simulink model "Concatenate9"  (R2017b)
settings: Solver=FixedStepAuto  StartTime=0.0  StopTime=0  FixedStep=0.1  MaxStep=1  RelTol=1e-3  EnableMultiTasking=on
settings Model: Creator=arnaud  LastModifiedBy=hbourbou
settings DataIOCC: LimitDataPoints=on  SaveFormat=Structure
settings OptimizationCC: LifeSpan=inf
settings DebuggingCC: SolverPrmCheckMsg=warning  SFUnexpectedBacktrackingDiag=warning  SFNoUnconditionalDefaultTransitionDiag=warning  SFExecutionAtInitializationDiag=none
settings HardwareCC: ProdBitPerPointer=32  ProdBitPerSizeT=32  ProdBitPerPtrDiffT=32  ProdLargestAtomicFloat=None  ProdIntDivRoundTo=Undefined  ProdEndianess=Unspecified  ProdWordSize=32  ProdHWDeviceType=32-bit Generic
settings ModelReferenceCC: PropagateSignalLabelsOutOfModel=off
settings CodeAppCC: StateflowObjectComments=on
settings GRTTargetCC: TargetLangStandard=C89/C90 (ANSI)  GeneratePreprocessorConditionals=Disable all
settings ConfigComp: CovMetricSettings=dw  CovHtmlReporting=on  CovSaveCumulativeToWorkspaceVar=on  CovSaveSingleToWorkspaceVar=on  CovExternalEMLEnable=off  CovSFcnEnable=off

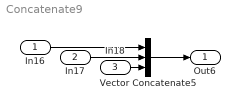
== system Concatenate9 ==
  In16 : Inport  OutDataTypeStr=double  PortDimensions=[5 2]
  In17 : Inport  Port=2  OutDataTypeStr=double  PortDimensions=[3 2]
  In18 : Inport  Port=3  OutDataTypeStr=double  PortDimensions=[1 2]
  Vector Concatenate5 : Concatenate  NumInputs=3  Mode=Multidimensional array
  Out6 : Outport
  wires:
  Vector Concatenate5/1 -> Out6/1
  In16/1 -> Vector Concatenate5/1
  In17/1 -> Vector Concatenate5/2
  In18/1 -> Vector Concatenate5/3
